simulink model "asd"  (R2017a)
settings: Solver=ode1  StartTime=0.0  StopTime=inf  FixedStep=0.002  RelTol=1e-3  EnableMultiTasking=on
PostLoadFcn:
  | qc_set_target_type(getConfigSet(bdroot, 'QUARC Default Target Configuration'));
values from neighbouring files (symbols this model uses):
  A_L = [0 1 0 0 0 0 ... (first row only)    [oppgave4c.m]    (also in oppgave4csiste.m)
  B_L = [0 0; 0 K_1; 0 0; K_2 0; 0 0; 0 0]    [oppgave4c.m]    (also in oppgave4csiste.m)
  C_L = [1 0 0 0 0 0 ... (first row only)    [oppgave4c.m]    (also in oppgave4csiste.m)
  Joystick_gain_x = 1    [oppgave4c.m]    (also in oppgave4csiste.m)
  Joystick_gain_y = -1    [oppgave4c.m]    (also in oppgave4csiste.m)
  K = lqr(A,B,Q,R)    [oppgave4c.m]    (also in oppgave4csiste.m)
  L = (place(A_L',C_L',poles))'    [oppgave4c.m]    (also in oppgave4csiste.m)
  P = eye(2)    [oppgave4c.m]
undefined symbols (not defined in the file or in its folder): HIL, qc_get_step_size
libraries: simulink_extras x12, quarc_library x4
settings Model: SimulationMode=external  ExtModeTrigDuration=5000  Creator=Rchan  LastModifiedBy=asgeirhu
settings SolverCC: PositivePriorityOrder=on
settings DataIOCC: LimitDataPoints=on  SaveFormat=Array  SignalLoggingSaveFormat=ModelDataLogs
settings OptimizationCC: ExpressionDepthLimit=2147483647  InitFltsAndDblsToZero=on  LifeSpan=inf
settings DebuggingCC: SaveWithParameterizedLinksMsg=none  UnderspecifiedInitializationDetection=Classic  MergeDetectMultiDrivingBlocksExec=none  SolverPrmCheckMsg=warning  MultiTaskDSMMsg=warning  MultiTaskCondExecSysMsg=none  FcnCallInpInsideContextMsg=warning  StateNameClashWarn=warning  SFUnexpectedBacktrackingDiag=warning  SFNoUnconditionalDefaultTransitionDiag=warning  SFExecutionAtInitializationDiag=none
settings HardwareCC: ProdBitPerPointer=32  ProdBitPerSizeT=32  ProdBitPerPtrDiffT=32  ProdLargestAtomicFloat=None  ProdIntDivRoundTo=Undefined  ProdEndianess=Unspecified  ProdWordSize=32  ProdHWDeviceType=32-bit Generic
settings ModelReferenceCC: PropagateSignalLabelsOutOfModel=off
settings RTWCC: SystemTargetFile=quarc_win64.tlc  TemplateMakefile=quarc_default_tmf  Description=QUARC Win64 Target
settings STFCustomTargetCC: TargetPreCompLibLocation=C:\PROGRA~3\QUARC\lib\2014a\win64\release  ConcurrentExecutionCompliant=on  GeneratePreprocessorConditionals=Disable all  CPPClassGenCompliant=on  SystemTargetFile=quarc_win64.tlc
settings GRTTargetCC: TargetPreCompLibLocation=C:\PROGRA~3\QUARC\lib\2014a\win64\release  TargetLangStandard=C89/C90 (ANSI)  ParMdlRefBuildCompliant=off  CompOptLevelCompliant=off  GeneratePreprocessorConditionals=Disable all  CombineOutputUpdateFcns=off  MatFileLogging=off  GRTInterface=on  UseToolchainInfoCompliant=off  ExtMode=on  ExtModeMexFile=quarc_comm
settings ConfigComp: CovMetricSettings=dw  CovHtmlReporting=on  CovSaveCumulativeToWorkspaceVar=on  CovSaveSingleToWorkspaceVar=on  CovExternalEMLEnable=off  CovSFcnEnable=off

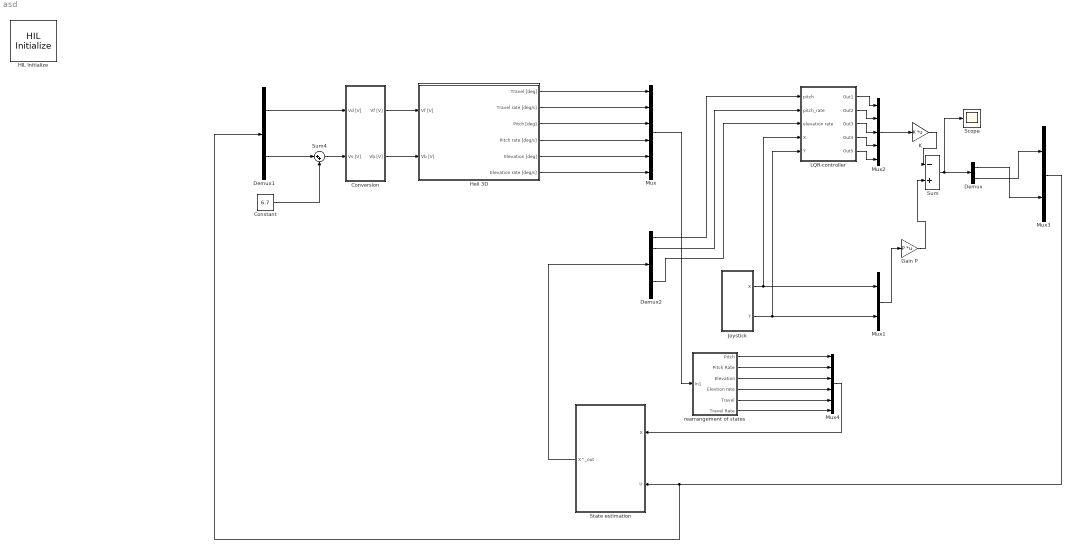
== system asd ==
  Constant : Constant  Value=6.7
  Conversion : Subsystem
  Demux : Demux  Outputs=2
  Demux1 : Demux  Outputs=2
  Demux2 : Demux  Outputs=6
  "Gain P " : Gain  Gain=P  Multiplication=Matrix(K*u)
  HIL Initialize : quarc_library/Data Acquisition/Generic/Configuration/HIL Initialize  Priority=-99  object_name=HIL-1  board_type=q8_usb  board_number=0  board_options=update_rate=normal;decimation=1  exclusive=off  active=off  hardware_clocks=[0:2]  clock_modes=[]  initial_clock_frequencies=[]  set_clock_params_at_start=off  set_clock_params_at_switch_in=off  set_clock_frequencies_at_start=off  set_clock_frequencies_at_switch_in=off  analog_input_channels=[0:7]  analog_input_maximums=10  analog_input_minimums=-10  set_analog_input_params_at_start=on  set_analog_input_params_at_switch_in=off  analog_output_channels=[0:7]  analog_output_maximums=10  analog_output_minimums=-10  initial_analog_outputs=[0]  final_analog_outputs=[0]  watchdog_analog_outputs=0  set_analog_output_params_at_start=on  set_analog_output_params_at_switch_in=off  set_analog_outputs_at_start=on  set_analog_outputs_at_switch_in=off  set_analog_outputs_at_terminate=on  set_analog_outputs_at_switch_out=off  set_analog_outputs_on_watchdog=off  digital_input_channels=[]  digital_output_channels=[]  digital_output_configuration=[]  initial_digital_outputs=[1]  final_digital_outputs=[1]  watchdog_digital_outputs=[1]  set_digital_output_params_at_start=off  set_digital_output_params_at_switch_in=off  set_digital_outputs_at_start=on  set_digital_outputs_at_switch_in=off  set_digital_outputs_at_terminate=on  set_digital_outputs_at_switch_out=off  set_digital_outputs_on_watchdog=off  encoder_channels=[0:7]  quadrature=[4]  encoder_filter_frequency=[]  initial_encoder_counts=[0]  set_encoder_params_at_start=on  set_encoder_params_at_switch_in=off  set_encoder_counts_at_start=on  set_encoder_counts_at_switch_in=off  pwm_channels=[0:7]  pwm_modes=0  pwm_frequency=99.532799999999995e6/4095  pwm_configuration=[0]  pwm_alignment=[0]  pwm_polarity=[1]  pwm_leading_deadband=[0]  pwm_trailing_deadband=[0]  initial_pwm_outputs=[0]  final_pwm_outputs=[0]  watchdog_pwm_outputs=[0]  set_pwm_params_at_start=on  set_pwm_params_at_switch_in=off  set_pwm_outputs_at_start=on  set_pwm_outputs_at_switch_in=off  set_pwm_outputs_at_terminate=on  set_pwm_outputs_at_switch_out=off  set_pwm_outputs_on_watchdog=off  other_output_channels=[]  initial_other_outputs=[]  final_other_outputs=[]  watchdog_other_outputs=[]  set_other_outputs_at_start=off  set_other_outputs_at_switch_in=off  set_other_outputs_at_terminate=off  set_other_outputs_at_switch_out=off  set_other_outputs_on_watchdog=off
  Heli 3D : Subsystem
  Joystick : Subsystem
  "K " : Gain  Gain=K  Multiplication=Matrix(K*u)
  LQR-controller : Subsystem
  Mux : Mux  Inputs=6
  Mux1 : Mux  Inputs=2
  Mux2 : Mux  Inputs=5
  Mux3 : Mux  Inputs=2
  Mux4 : Mux  Inputs=6
  Scope : Scope
  "State estimation " : Subsystem
  Sum : Sum  Inputs=-+
  Sum4 : Sum  Inputs=|++
  rearrangement of states : Subsystem
  wires:
  Conversion/2(Vb [V]) -> Heli 3D/2(Vb [V])
  Heli 3D/1(Travel [deg]) -> Mux/1
  Heli 3D/2(Travel rate [deg/s]) -> Mux/2
  Heli 3D/3(Pitch [deg]) -> Mux/3
  Heli 3D/6(Elevation rate [deg/s]) -> Mux/6
  Joystick/1(X) -> Mux1/1, LQR-controller/4(X)
  Joystick/2(Y) -> LQR-controller/5(Y), Mux1/2
  Mux1/1 -> "Gain P "/1
  Mux2/1 -> "K "/1
  "K "/1 -> Sum/1
  "Gain P "/1 -> Sum/2
  Sum/1 -> Demux/1, Scope/1
  Demux/2 -> Mux3/1
  Conversion/1(Vf [V]) -> Heli 3D/1(Vf [V])
  Demux1/1 -> Conversion/1(Vd [V])
  Mux3/1 -> Demux1/1, "State estimation "/2("U ")
  Mux/1 -> rearrangement of states/1(In1)
  rearrangement of states/1("Pitch ") -> Mux4/1
  rearrangement of states/2(Pitch Rate) -> Mux4/2
  rearrangement of states/3("Elevation ") -> Mux4/3
  rearrangement of states/4(Elevtion rate) -> Mux4/4
  rearrangement of states/5(Travel) -> Mux4/5
  rearrangement of states/6(Travel Rate) -> Mux4/6
  Mux4/1 -> "State estimation "/1(X)
  LQR-controller/1(Out1) -> Mux2/1
  LQR-controller/2(Out2) -> Mux2/2
  LQR-controller/3(Out3) -> Mux2/3
  LQR-controller/4(Out4) -> Mux2/4
  LQR-controller/5(Out5) -> Mux2/5
  Heli 3D/4(Pitch rate [deg/s]) -> Mux/4
  Heli 3D/5(Elevation [deg]) -> Mux/5
  Sum4/1 -> Conversion/2(Vs [V])
  Demux/1 -> Mux3/2
  "State estimation "/1("X^_out ") -> Demux2/1
  Demux1/2 -> Sum4/1
  Constant/1 -> Sum4/2
  Demux2/1 -> LQR-controller/1("pitch ")
  Demux2/2 -> LQR-controller/2(pitch_rate)
  Demux2/5 -> LQR-controller/3("elevation rate ")

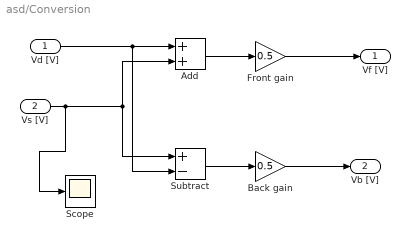
== system asd/Conversion ==
  Vd [V] : Inport
  Vs [V] : Inport  Port=2
  Add : Sum
  Back gain : Gain  Gain=0.5
  Front gain : Gain  Gain=0.5
  Scope : Scope
  Subtract : Sum  Inputs=+-
  Vf [V] : Outport
  Vb [V] : Outport  Port=2
  wires:
  Vd [V]/1 -> Subtract/2, Add/1
  Vs [V]/1 -> Scope/1, Subtract/1, Add/2
  Subtract/1 -> Back gain/1
  Back gain/1 -> Vb [V]/1
  Add/1 -> Front gain/1
  Front gain/1 -> Vf [V]/1

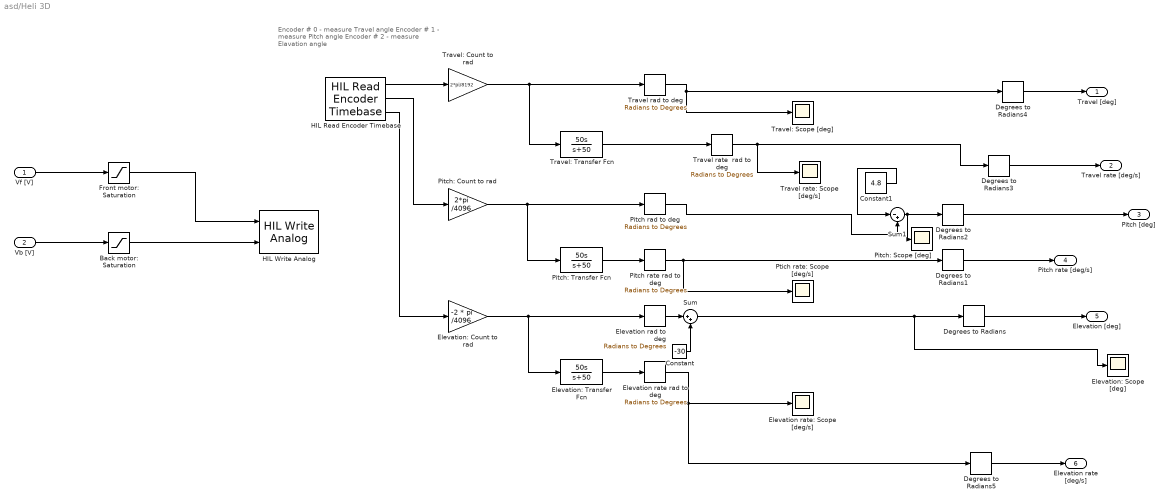
== system asd/Heli 3D ==
  note: Encoder # 0 - measure Travel angle
      | Encoder # 1 - measure Pitch angle
      | Encoder # 2 - measure Elavation angle
  Vf [V] : Inport
  Vb [V] : Inport  Port=2
  Back motor: Saturation : Saturate  UpperLimit=5  LowerLimit=-5
  Constant : Constant  Value=-30
  Constant1 : Constant  Value=4.8
  Degrees to Radians{,1..5} (6 alike) : simulink_extras/Transformations/Degrees to Radians
  Elevation rad to deg : simulink_extras/Transformations/Radians to Degrees
  Elevation rate rad to deg : simulink_extras/Transformations/Radians to Degrees
  Elevation rate: Scope [deg/s] : Scope
  Elevation: Count to rad : Gain  Gain=-2 * pi /4096
  Elevation: Scope [deg] : Scope
  Elevation: Transfer Fcn : TransferFcn  Numerator=[50 0]  Denominator=[1 50]
  Front motor: Saturation : Saturate  UpperLimit=5  LowerLimit=-5
  HIL Read Encoder Timebase : quarc_library/Data Acquisition/Generic/Timebases/HIL Read Encoder Timebase  object_name=HIL-1  clock=0  channels=[0:2]  samples_in_buffer=max(ceil(1/qc_get_step_size), 1)  active=on  vector_output=off  data_type_mode=Inherit via back propagation  data_type=double
  HIL Write Analog : quarc_library/Data Acquisition/Generic/Immediate I//O/HIL Write Analog  object_name=HIL-1  channels=[0:1]  sample_time=-1  active=off  vector_input=off
  Pitch rad to deg : simulink_extras/Transformations/Radians to Degrees
  Pitch rate rad to deg : simulink_extras/Transformations/Radians to Degrees
  Pitch: Count to rad : Gain  Gain=2*pi /4096
  Pitch: Scope [deg] : Scope
  Pitch: Transfer Fcn : TransferFcn  Numerator=[50 0]  Denominator=[1 50]
  Ptich rate: Scope [deg/s] : Scope
  Sum : Sum  Inputs=|++
  Sum1 : Sum  Inputs=|-+
  Travel rad to deg : simulink_extras/Transformations/Radians to Degrees
  Travel rate  rad to deg : simulink_extras/Transformations/Radians to Degrees
  Travel rate: Scope [deg/s] : Scope
  Travel: Count to rad : Gain  Gain=2*pi/8192
  Travel: Scope [deg] : Scope
  Travel: Transfer Fcn : TransferFcn  Numerator=[50 0]  Denominator=[1 50]
  Travel [deg] : Outport
  Travel rate [deg/s] : Outport  Port=2
  Pitch [deg] : Outport  Port=3
  Pitch rate [deg/s] : Outport  Port=4
  Elevation [deg] : Outport  Port=5
  Elevation rate [deg/s] : Outport  Port=6
  wires:
  HIL Read Encoder Timebase/1 -> Travel: Count to rad/1
  HIL Read Encoder Timebase/2 -> Pitch: Count to rad/1
  HIL Read Encoder Timebase/3 -> Elevation: Count to rad/1
  Travel: Count to rad/1 -> Travel: Transfer Fcn/1, Travel rad to deg/1
  Travel: Transfer Fcn/1 -> Travel rate  rad to deg/1
  Pitch: Count to rad/1 -> Pitch: Transfer Fcn/1, Pitch rad to deg/1
  Pitch: Transfer Fcn/1 -> Pitch rate rad to deg/1
  Elevation: Count to rad/1 -> Elevation: Transfer Fcn/1, Elevation rad to deg/1
  Elevation: Transfer Fcn/1 -> Elevation rate rad to deg/1
  Travel rad to deg/1 -> Travel: Scope [deg]/1, Degrees to Radians4/1
  Travel rate  rad to deg/1 -> Travel rate: Scope [deg/s]/1, Degrees to Radians3/1
  Pitch rad to deg/1 -> Sum1/2
  Pitch rate rad to deg/1 -> Ptich rate: Scope [deg/s]/1, Degrees to Radians1/1
  Vf [V]/1 -> Front motor: Saturation/1
  Vb [V]/1 -> Back motor: Saturation/1
  Front motor: Saturation/1 -> HIL Write Analog/1
  Back motor: Saturation/1 -> HIL Write Analog/2
  Elevation rate rad to deg/1 -> Elevation rate: Scope [deg/s]/1, Degrees to Radians5/1
  Constant/1 -> Sum/2
  Elevation rad to deg/1 -> Sum/1
  Sum/1 -> Degrees to Radians/1, Elevation: Scope [deg]/1
  Degrees to Radians/1 -> Elevation [deg]/1
  Degrees to Radians1/1 -> Pitch rate [deg/s]/1
  Degrees to Radians2/1 -> Pitch [deg]/1
  Degrees to Radians3/1 -> Travel rate [deg/s]/1
  Degrees to Radians4/1 -> Travel [deg]/1
  Degrees to Radians5/1 -> Elevation rate [deg/s]/1
  Constant1/1 -> Sum1/1
  Sum1/1 -> Degrees to Radians2/1, Pitch: Scope [deg]/1

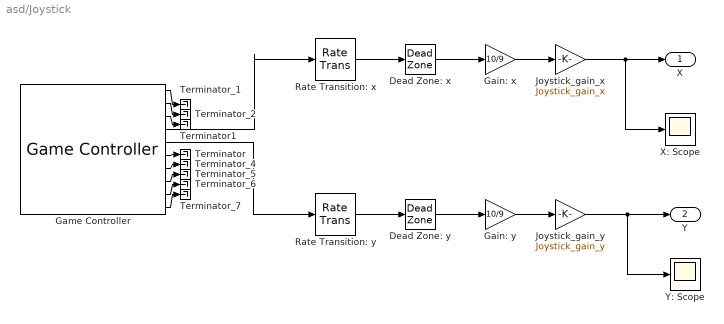
== system asd/Joystick ==
  Dead Zone: x : DeadZone  LowerValue=-0.1  UpperValue=0.1  SaturateOnIntegerOverflow=on
  Dead Zone: y : DeadZone  LowerValue=-0.1  UpperValue=0.1  SaturateOnIntegerOverflow=on
  Gain: x : Gain  Gain=10/9
  Gain: y : Gain  Gain=10/9
  Game Controller : quarc_library/Devices/Peripherals/Target/Game Controller  controller=1  buffer_size=12  deadzone=[]  saturation=[]  sample_time=max(qc_get_step_size, 0.01)  auto_center=off  enabled=on
  Joystick_gain_x : Gain  Gain=Joystick_gain_x
  Joystick_gain_y : Gain  Gain=Joystick_gain_y
  Rate Transition: x : RateTransition
  Rate Transition: y : RateTransition
  Terminator : Terminator
  Terminator1 : Terminator
  Terminator_{1..2,4..7} (6 alike) : Terminator
  X: Scope : Scope
  Y: Scope : Scope
  X : Outport
  Y : Outport  Port=2
  wires:
  Rate Transition: y/1 -> Dead Zone: y/1
  Rate Transition: x/1 -> Dead Zone: x/1
  Game Controller/5 -> Rate Transition: y/1
  Game Controller/4 -> Rate Transition: x/1
  Game Controller/1 -> Terminator_1/1
  Game Controller/2 -> Terminator_2/1
  Game Controller/7 -> Terminator_4/1
  Game Controller/8 -> Terminator_5/1
  Game Controller/9 -> Terminator_6/1
  Game Controller/10 -> Terminator_7/1
  Game Controller/3 -> Terminator1/1
  Game Controller/6 -> Terminator/1
  Dead Zone: x/1 -> Gain: x/1
  Dead Zone: y/1 -> Gain: y/1
  Gain: x/1 -> Joystick_gain_x/1
  Gain: y/1 -> Joystick_gain_y/1
  Joystick_gain_x/1 -> X/1, X: Scope/1
  Joystick_gain_y/1 -> Y: Scope/1, Y/1

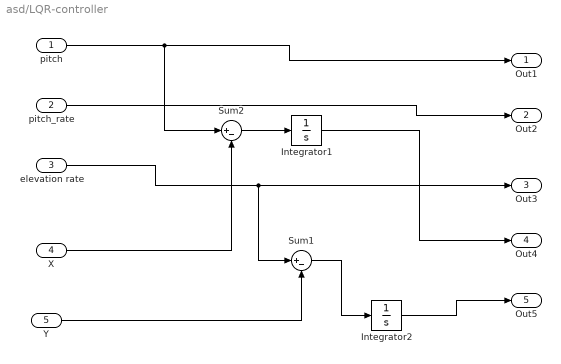
== system asd/LQR-controller ==
  "pitch " : Inport
  pitch_rate : Inport  Port=2
  "elevation rate " : Inport  Port=3
  X : Inport  Port=4
  Y : Inport  Port=5
  Integrator1 : Integrator
  Integrator2 : Integrator
  Sum1 : Sum  Inputs=|+-
  Sum2 : Sum  Inputs=|+-
  Out1 : Outport
  Out2 : Outport  Port=2
  Out3 : Outport  Port=3
  Out4 : Outport  Port=4
  Out5 : Outport  Port=5
  wires:
  "pitch "/1 -> Sum2/1, Out1/1
  X/1 -> Sum2/2
  Sum2/1 -> Integrator1/1
  Integrator1/1 -> Out4/1
  pitch_rate/1 -> Out2/1
  "elevation rate "/1 -> Sum1/1, Out3/1
  Y/1 -> Sum1/2
  Sum1/1 -> Integrator2/1
  Integrator2/1 -> Out5/1

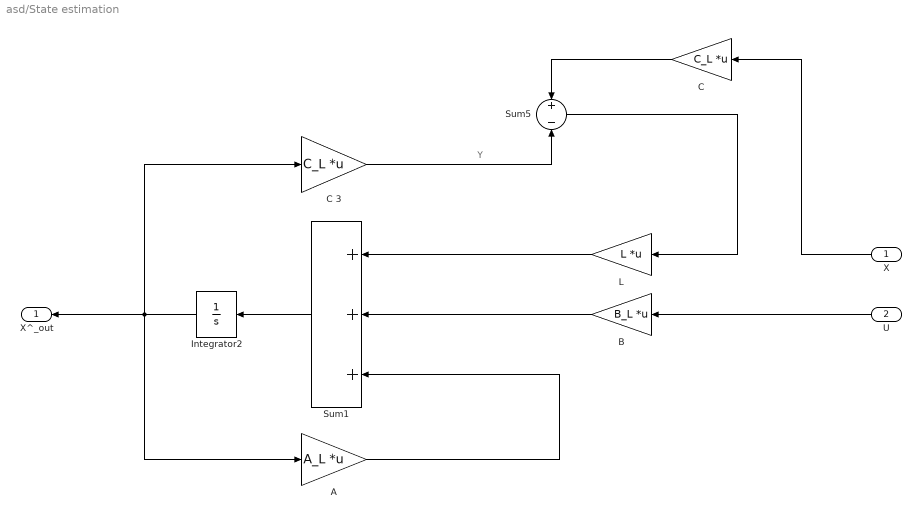
== system asd/State estimation  ==
  note: Y
  X : Inport
  "U " : Inport  Port=2
  "A " : Gain  Gain=A_L  Multiplication=Matrix(K*u)
  "B " : Gain  Gain=B_L  Multiplication=Matrix(K*u)
  "C " : Gain  Gain=C_L  Multiplication=Matrix(K*u)
  C 3 : Gain  Gain=C_L  Multiplication=Matrix(K*u)
  Integrator2 : Integrator
  "L " : Gain  Gain=L  Multiplication=Matrix(K*u)
  Sum1 : Sum  Inputs=+++
  Sum5 : Sum  Inputs=+|-
  "X^_out " : Outport
  wires:
  "A "/1 -> Sum1/3
  C 3/1 -> Sum5/2
  "B "/1 -> Sum1/2
  Sum5/1 -> "L "/1
  "U "/1 -> "B "/1
  Integrator2/1 -> "A "/1, C 3/1, "X^_out "/1
  Sum1/1 -> Integrator2/1
  "C "/1 -> Sum5/1
  X/1 -> "C "/1
  "L "/1 -> Sum1/1

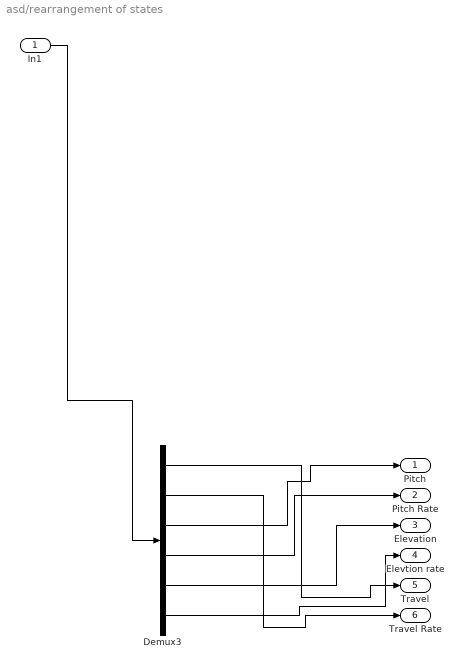
== system asd/rearrangement of states ==
  In1 : Inport
  Demux3 : Demux  Outputs=6
  "Pitch " : Outport
  Pitch Rate : Outport  Port=2
  "Elevation " : Outport  Port=3
  Elevtion rate : Outport  Port=4
  Travel : Outport  Port=5
  Travel Rate : Outport  Port=6
  wires:
  Demux3/5 -> "Elevation "/1
  Demux3/1 -> Travel/1
  Demux3/3 -> "Pitch "/1
  Demux3/4 -> Pitch Rate/1
  In1/1 -> Demux3/1
  Demux3/2 -> Travel Rate/1
  Demux3/6 -> Elevtion rate/1
